simulink model "NL_valve_MSAM_2"  (Simulink 7.8)
settings: Solver=ode45  StartTime=0.0  StopTime=time_span  RelTol=1e-3
values from neighbouring files (symbols this model uses):
  samp_time = p.simulation.samp_time    [MSA_Controller.m]    (also in MSA_Controller_NL_valve.m)
undefined symbols (not defined in the file or in its folder): outstr, p
libraries: simulink_need_slupdate x1
settings Model: Creator=KushalSahare  LastModifiedBy=Kushal

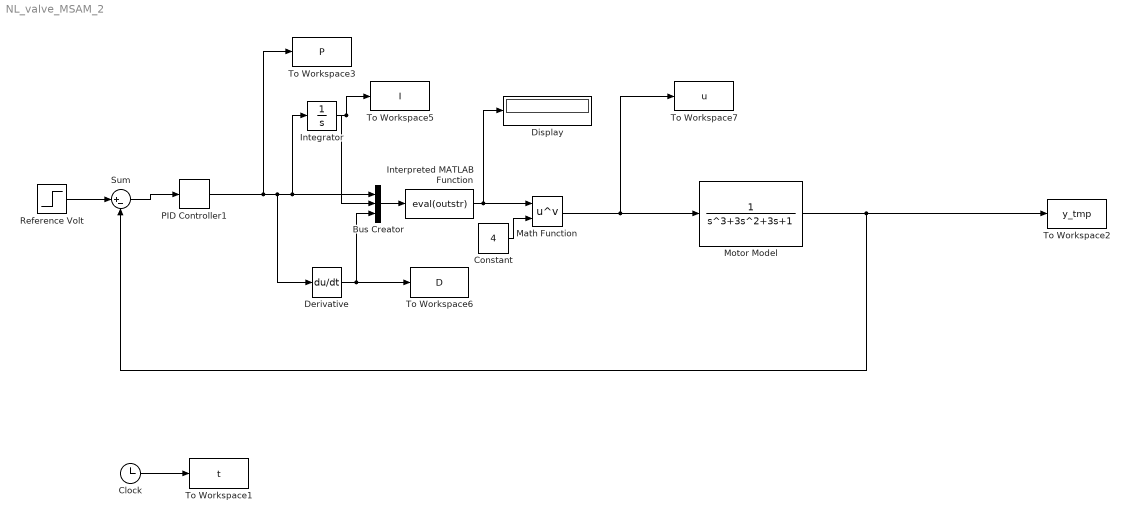
== system NL_valve_MSAM_2 ==
  Bus Creator : BusCreator  Inputs=3
  Clock : Clock
  Constant : Constant  Value=4
  Derivative : Derivative
  Display : Display
  Integrator : Integrator
  Interpreted MATLAB Function : MATLABFcn  MATLABFcn=eval(outstr)  OutputSignalType=real
  Math Function : Math  Operator=pow  SaturateOnIntegerOverflow=on
  Motor Model : TransferFcn  Numerator=1  Denominator=[1, 3, 3, 1]
  PID Controller1 : simulink_need_slupdate/PID Controller  P=1  I=0  D=0
  Reference Volt : Step  Time=0  After=p.simulation.Cm  SampleTime=0
  Sum : Sum  Inputs=|+-
  To Workspace1 : ToWorkspace  VariableName=t  SampleTime=samp_time  SaveFormat=Array
  To Workspace2 : ToWorkspace  VariableName=y_tmp  SampleTime=samp_time  SaveFormat=Array
  To Workspace3 : ToWorkspace  VariableName=P  SampleTime=samp_time  SaveFormat=Array
  To Workspace5 : ToWorkspace  VariableName=I  SampleTime=samp_time  SaveFormat=Array
  To Workspace6 : ToWorkspace  VariableName=D  SampleTime=samp_time  SaveFormat=Array
  To Workspace7 : ToWorkspace  VariableName=u  SampleTime=samp_time  SaveFormat=Array
  wires:
  Motor Model/1 -> Sum/2, To Workspace2/1
  Reference Volt/1 -> Sum/1
  Math Function/1 -> Motor Model/1, To Workspace7/1
  Clock/1 -> To Workspace1/1
  Derivative/1 -> Bus Creator/3, To Workspace6/1
  Integrator/1 -> To Workspace5/1, Bus Creator/2
  Bus Creator/1 -> Interpreted MATLAB Function/1
  Interpreted MATLAB Function/1 -> Math Function/1, Display/1
  Constant/1 -> Math Function/2
  PID Controller1/1 -> To Workspace3/1, Derivative/1, Bus Creator/1, Integrator/1
  Sum/1 -> PID Controller1/1
